simulink model "rotational_wheel_dynamics"  (R2024a)
settings: Solver=ode45  StartTime=0.0  StopTime=10.0  RelTol=1e-3
values from neighbouring files (symbols this model uses):
  f0 = 0.009    [assignment_2.m]
  f2 = 6.5*10^(-6)    (= 6.5e-06)    [assignment_2.m]
  Ir = 1.46    [assignment_2.m]
  R = 0.3488    [assignment_2.m]
  velstart = 3    [assignment_2.m]
settings Model: Creator=fjmo  LastModifiedBy=fjmo

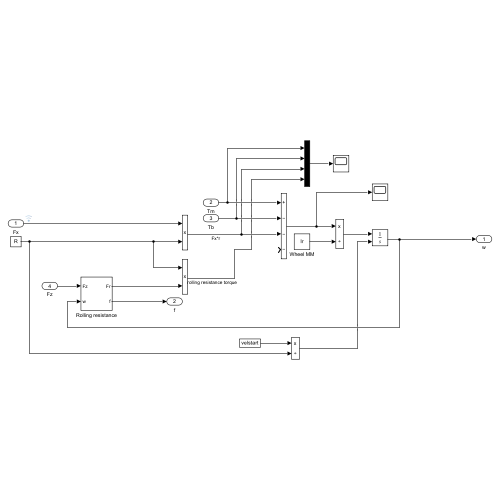
[thumbnail: Simulink's stored preview of the top-level diagram]
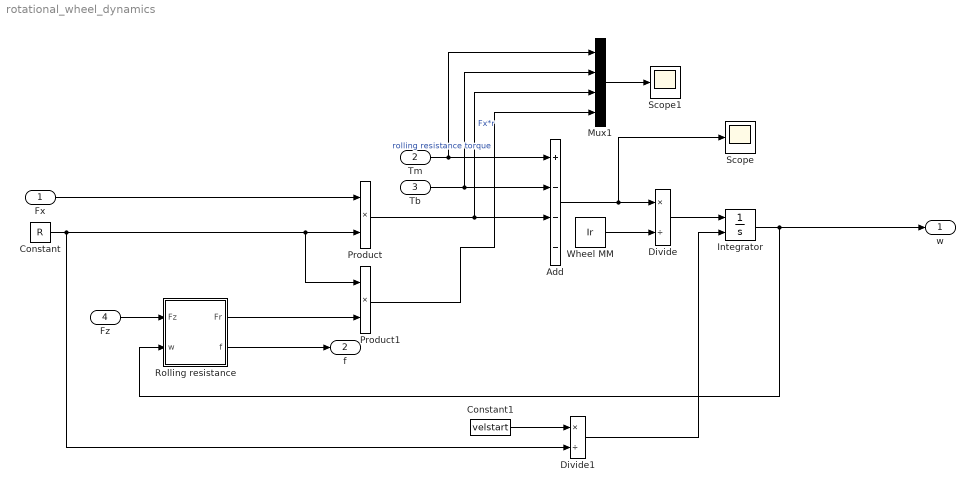
== system rotational_wheel_dynamics ==
  Fx : Inport
  Tm : Inport  Port=2
  Tb : Inport  Port=3
  Fz : Inport  Port=4
  Add : Sum  Inputs=+---
  Constant : Constant  Value=R
  Constant1 : Constant  Value=velstart
  Divide : Product  Inputs=*/
  Divide1 : Product  Inputs=*/
  Integrator : Integrator  InitialConditionSource=external
  Mux1 : Mux
  Product : Product
  Product1 : Product
  Rolling resistance : Subsystem
  Scope : Scope
  Scope1 : Scope
  Wheel MM : Constant  Value=Ir
  w : Outport
  f : Outport  Port=2
  wires:
  Tm/1 -> Mux1/1, Add/1
  Tb/1 -> Mux1/2, Add/2
  Constant/1 -> Product/2, Product1/1, Divide1/2
  Product/1 -> Mux1/3, Add/3  "Fx*r"
  Add/1 -> Scope/1, Divide/1
  Wheel MM/1 -> Divide/2
  Divide/1 -> Integrator/1
  Divide1/1 -> Integrator/2
  Mux1/1 -> Scope1/1
  Constant1/1 -> Divide1/1
  Fz/1 -> Rolling resistance/1(Fz)
  Product1/1 -> Mux1/4  "rolling resistance torque"
  Rolling resistance/1(Fr) -> Product1/2
  Rolling resistance/2(f) -> f/1
  Integrator/1 -> w/1, Rolling resistance/2(w)
  Fx/1 -> Product/1

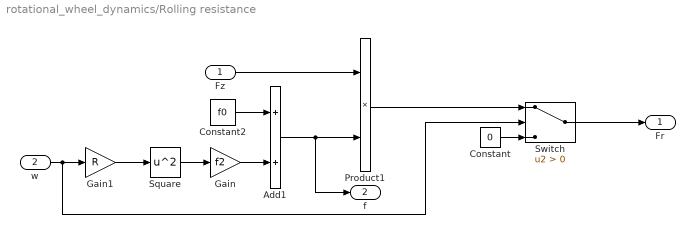
== system rotational_wheel_dynamics/Rolling resistance ==
  Fz : Inport
  w : Inport  Port=2
  Add1 : Sum
  Constant : Constant  Value=0
  Constant2 : Constant  Value=f0
  Gain : Gain  Gain=f2
  Gain1 : Gain  Gain=R
  Product1 : Product
  Square : Math  Operator=square
  Switch : Switch  Criteria=u2 > Threshold  SaturateOnIntegerOverflow=off  InputSameDT=off
  Fr : Outport
  f : Outport  Port=2
  wires:
  Constant2/1 -> Add1/1
  Square/1 -> Gain/1
  Gain1/1 -> Square/1
  Fz/1 -> Product1/1
  w/1 -> Switch/2, Gain1/1
  Gain/1 -> Add1/2
  Add1/1 -> f/1, Product1/2
  Constant/1 -> Switch/3
  Switch/1 -> Fr/1
  Product1/1 -> Switch/1
